simulink model "synch"  (Simulink 4.00)
settings: Solver=ode45  StartTime=0.0  StopTime=25.0  RelTol=1e-3
InitFcn:
  | clear functions
libraries: truetime x1, simulink3 x1
settings Model: Creator=user  LastModifiedBy=anton  SaveTime=off  SaveOutput=off  ExtModeAutoUpdateStatusClock=off

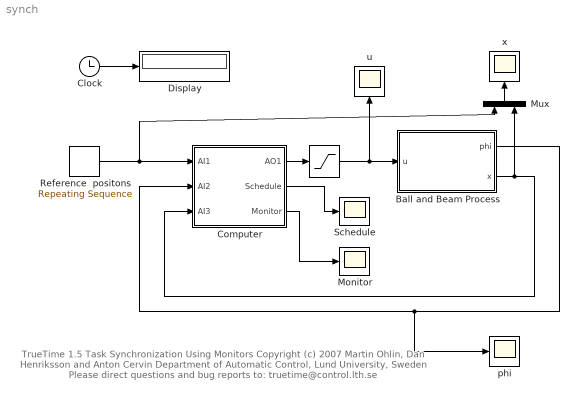
== system synch ==
  note: TrueTime 1.5  Task Synchronization Using Monitors
      | Copyright (c) 2007
      | Martin Ohlin, Dan Henriksson and Anton Cervin
      | Department of Automatic Control, Lund University, Sweden
      | Please direct questions and bug reports to:  truetime@control.lth.se
  " " : Saturate  UpperLimit=10  LowerLimit=-10  LinearizeAsGain=on
  Ball and Beam Process : Subsystem
      settings: RTWFcnNameOpts=Auto  RTWFileNameOpts=Auto
  Clock : Clock
      settings: DisplayTime=off  Decimation=10
  Computer : Subsystem
      settings: RTWFcnNameOpts=Auto  RTWFileNameOpts=Auto
  Display : Display
      settings: Format=short
  Monitor : Scope
      settings: TickLabels=on  TimeRange=25  YMin=0.8  YMax=2.7  SaveToWorkspace=off  SaveName=ScopeData4  DataFormat=Array  MaxDataPoints=5000
  Mux : Mux  Orientation=up  Inputs=2
  Reference  positons : simulink3/Sources/Repeating Sequence  rep_seq_t=[0 1 1 5 5 9 9 13 13 17 17 21 21 25]  rep_seq_y=[0 0 5 5 -3 -3 8 8 0 0 2 2 -7 -7]
  Schedule : Scope
      settings: TickLabels=on  TimeRange=25  YMin=0.8  YMax=2.7  SaveToWorkspace=off  DataFormat=Array  MaxDataPoints=5000
  phi : Scope
      settings: TimeRange=25  YMin=-8  YMax=10  SaveToWorkspace=off  SaveName=ScopeData  MaxDataPoints=5000
  u : Scope
      settings: Orientation=up  TimeRange=25  YMin=-10  YMax=10  SaveToWorkspace=off  SaveName=ScopeData3  MaxDataPoints=5000
  x : Scope
      settings: Orientation=up  TimeRange=25  YMin=-8  YMax=10  SaveToWorkspace=off  SaveName=ScopeData2  MaxDataPoints=5000
  wires:
  Clock/1 -> Display/1
  Ball and Beam Process/2(x) -> Mux/2, Computer/3(AI3)
  Ball and Beam Process/1(phi) -> Computer/2(AI2), phi/1
  Reference  positons/1 -> Computer/1(AI1), Mux/1
  Computer/1(AO1) -> " "/1
  Mux/1 -> x/1
  Computer/2(Schedule) -> Schedule/1
  Computer/3(Monitor) -> Monitor/1
  " "/1 -> u/1, Ball and Beam Process/1(u)

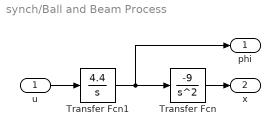
== system synch/Ball and Beam Process ==
  u : Inport  Port=1  LatchInput=off
  Transfer Fcn : TransferFcn  Numerator=[-9]  Denominator="[1  0 0]"  AbsoluteTolerance=auto  Realization=auto
  Transfer Fcn1 : TransferFcn  Numerator=4.4  Denominator=[1 0]  AbsoluteTolerance=auto  Realization=auto
  phi : Outport  Port=1
  x : Outport  Port=2
  wires:
  u/1 -> Transfer Fcn1/1
  Transfer Fcn1/1 -> phi/1, Transfer Fcn/1
  Transfer Fcn/1 -> x/1

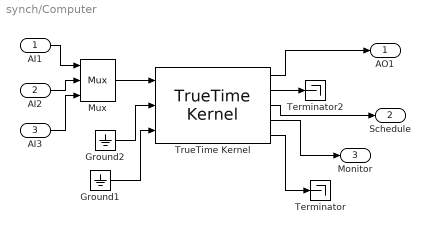
== system synch/Computer ==
  AI1 : Inport  Port=1  LatchInput=off
  AI2 : Inport  Port=2  LatchInput=off
  AI3 : Inport  Port=3  LatchInput=off
  Ground1 : Ground
  Ground2 : Ground
  Mux : Mux  Inputs=3
      settings: DisplayOption=none
  Terminator : Terminator
  Terminator2 : Terminator
  TrueTime Kernel : truetime/TrueTime Kernel  sfun=synch_init  args=0  battery=off  clockdrift=0  clockoffset=0
  AO1 : Outport  Port=1
  Schedule : Outport  Port=2
  Monitor : Outport  Port=3
  wires:
  AI1/1 -> Mux/1
  AI2/1 -> Mux/2
  TrueTime Kernel/2 -> Terminator2/1
  Ground2/1 -> TrueTime Kernel/2
  AI3/1 -> Mux/3
  Mux/1 -> TrueTime Kernel/1
  Ground1/1 -> TrueTime Kernel/3
  TrueTime Kernel/4 -> Monitor/1
  TrueTime Kernel/3 -> Schedule/1
  TrueTime Kernel/1 -> AO1/1
  TrueTime Kernel/5 -> Terminator/1
